simulink model "Schema_inversione_cinematica_con_pseudo_inversa_Jacobiano"  (R2023a)
settings: Solver=VariableStepAuto  StartTime=0.0  StopTime=113  RelTol=1e-3
values from neighbouring files (symbols this model uses):
  a1 = 0.5    [Progetto_FoR.m]
  d0 = 1    [Progetto_FoR.m]
  K0 = 0    [Progetto_FoR.m]
  K_pinv = diag(k_pinv)    [Progetto_FoR.m]
  q0 = [0 pi/2 0 pi/2]    [Progetto_FoR.m]
  Tc = 0.001    [Progetto_FoR.m]
undefined symbols (not defined in the file or in its folder): DiscIntNeverNeededParam
settings Model: Creator=panto  LastModifiedBy=panto

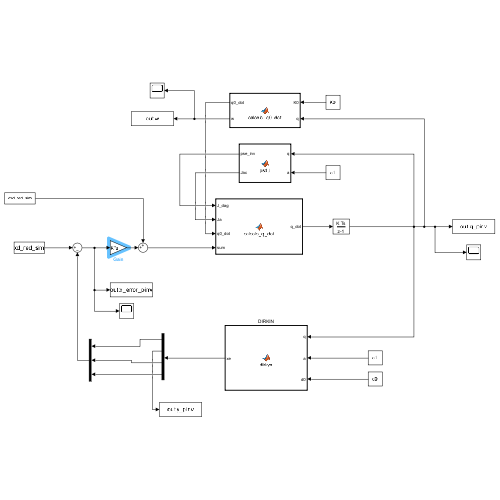
[thumbnail: Simulink's stored preview of the top-level diagram]
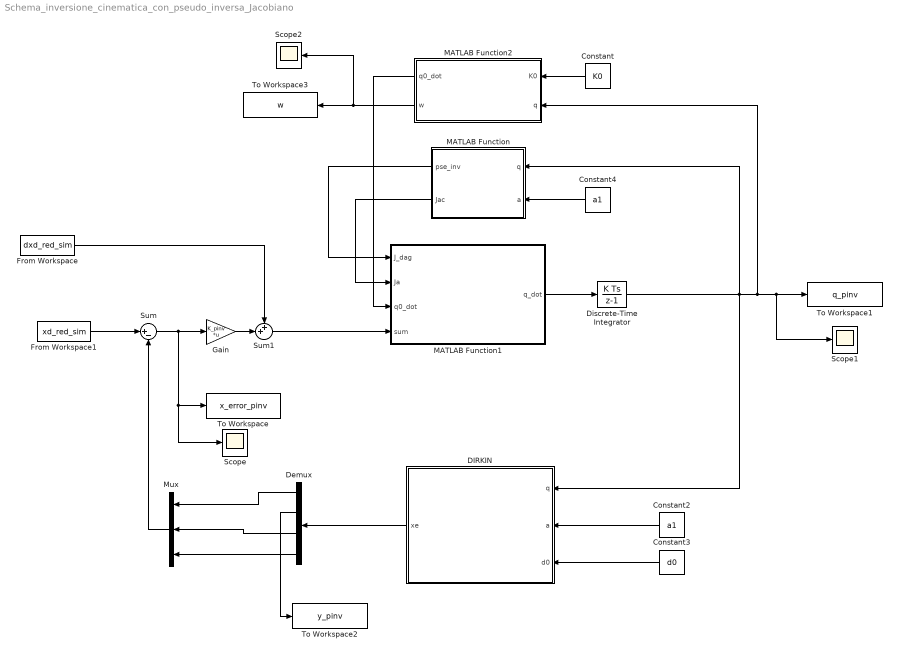
== system Schema_inversione_cinematica_con_pseudo_inversa_Jacobiano ==
  Constant : Constant  Value=K0
  Constant2 : Constant  Value=a1
  Constant3 : Constant  Value=d0
  Constant4 : Constant  Value=a1
  DIRKIN : MATLAB Function  TreatAsAtomicUnit=on
  Demux : Demux
  Discrete-Time Integrator : DiscreteIntegrator  InitialCondition=q0'  SampleTime=Tc  ICPrevOutput=DiscIntNeverNeededParam  ICPrevScaledInput=DiscIntNeverNeededParam
  From Workspace : FromWorkspace  VariableName=dxd_red_sim  SampleTime=Tc
  From Workspace1 : FromWorkspace  VariableName=xd_red_sim  SampleTime=Tc
  Gain : Gain  Gain=K_pinv  Multiplication=Matrix(K*u)
  MATLAB Function : MATLAB Function  TreatAsAtomicUnit=on
  MATLAB Function1 : MATLAB Function  TreatAsAtomicUnit=on
  MATLAB Function2 : MATLAB Function  TreatAsAtomicUnit=on
  Mux : Mux  Inputs=3
  Scope : Scope
  Scope1 : Scope
  Scope2 : Scope
  Sum : Sum  Inputs=|+-
  Sum1 : Sum  Inputs=++|
  To Workspace : ToWorkspace  VariableName=x_error_pinv  SampleTime=Tc
      settings: Save2DSignal=2-D array (concatenate along first dimension)
  To Workspace1 : ToWorkspace  VariableName=q_pinv  SampleTime=-1
      settings: Save2DSignal=2-D array (concatenate along first dimension)
  To Workspace2 : ToWorkspace  VariableName=y_pinv  SampleTime=-1
      settings: Save2DSignal=2-D array (concatenate along first dimension)
  To Workspace3 : ToWorkspace  VariableName=w  SampleTime=Tc
      settings: Save2DSignal=2-D array (concatenate along first dimension)
  wires:
  Constant2/1 -> DIRKIN/2(a)
  Constant3/1 -> DIRKIN/3(d0)
  From Workspace/1 -> Sum1/1
  Sum/1 -> To Workspace/1, Scope/1, Gain/1
  Gain/1 -> Sum1/2
  Constant4/1 -> MATLAB Function/2(a)
  Discrete-Time Integrator/1 -> DIRKIN/1(q), MATLAB Function/1(q), MATLAB Function2/2(q), Scope1/1, To Workspace1/1
  From Workspace1/1 -> Sum/1
  DIRKIN/1(xe) -> Demux/1
  Demux/1 -> Mux/1
  Demux/4 -> Mux/3
  Demux/3 -> Mux/2
  Mux/1 -> Sum/2
  Demux/2 -> To Workspace2/1
  MATLAB Function/1(pse_inv) -> MATLAB Function1/1(J_dag)
  MATLAB Function1/1(q_dot) -> Discrete-Time Integrator/1
  Sum1/1 -> MATLAB Function1/4(sum)
  MATLAB Function/2(Jac) -> MATLAB Function1/2(Ja)
  MATLAB Function2/1(q0_dot) -> MATLAB Function1/3(q0_dot)
  Constant/1 -> MATLAB Function2/1(K0)
  MATLAB Function2/2(w) -> Scope2/1, To Workspace3/1

== matlab function Schema_inversione_cinematica_con_pseudo_inversa_Jacobiano/DIRKIN ==
  data: q input; xe output; a input; d0 input
function xe = dirkyn(q, a, d0)
  xe = zeros(4,1);
    xe = [a*cos(q(1)+q(2))+a*cos(q(1));
        a*sin(q(1)+q(2))+a*sin(q(1));
        d0-q(3);
        q(1)+q(2)-q(4)];
end

== matlab function Schema_inversione_cinematica_con_pseudo_inversa_Jacobiano/MATLAB Function ==
  data: q input; pse_inv output; a input; Jac output
function [pse_inv,Jac] = psdJ(q,a)

%Levo la seconda riga perché ho deciso di rilassare la componente y
   
    Ja = zeros(3,4);
    Ja = [-a*sin(q(1)+q(2))-a*sin(q(1)) -a*sin(q(1)+q(2)) 0 0;
        0 0 -1 0;
        1 1 0 -1];

    J_dag = Ja'/(Ja*Ja');

    pse_inv = J_dag;
    Jac = Ja;

end

== matlab function Schema_inversione_cinematica_con_pseudo_inversa_Jacobiano/MATLAB Function1 ==
  data: J_dag input; Ja input; q_dot output; q0_dot input; sum input
function q_dot = calcolo_q_dot(J_dag,Ja,q0_dot,sum)
%sum = xd_dot+Ke

I = eye(4); %questo perchè J_dag J è una matrice 4x4

q_dot = J_dag*sum +(I-J_dag*Ja)*q0_dot;

end

== matlab function Schema_inversione_cinematica_con_pseudo_inversa_Jacobiano/MATLAB Function2 ==
  data: K0 input; q0_dot output; q input; w output
function [q0_dot,w] = calcolo_q0_dot(K0,q)

w = (sin(q(2)))^2;
der_w = sin(2*q(2)); %la derivata di sin^2(q) è 2cos(q)sin(q) = sin(2q)

q0_dot = [0; K0*(der_w)'; 0;0];

end
